simulink model "ModID_b2_R2018A"  (R2018b)
settings: Solver=VariableStepAuto  StartTime=0.0  StopTime=10.0  RelTol=1e-3
undefined symbols (not defined in the file or in its folder): par
settings Model: Creator=janneke  LastModifiedBy=janneke

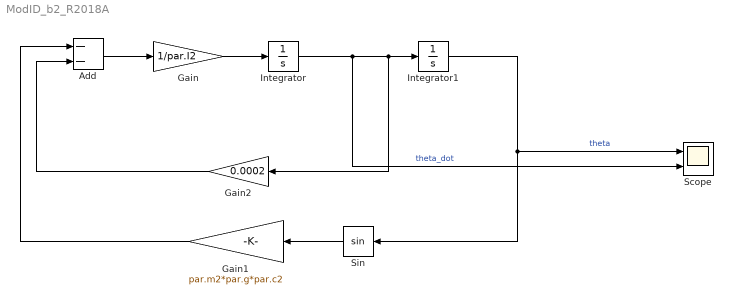
== system ModID_b2_R2018A ==
  Add : Sum  Inputs=--
  Gain : Gain  Gain=1/par.I2
  Gain1 : Gain  Gain=par.m2*par.g*par.c2
  Gain2 : Gain  Gain=0.0002
  Integrator : Integrator
  Integrator1 : Integrator  InitialCondition=-pi/2
  Scope : Scope  NumInputPorts=2
  Sin : Trigonometry
  wires:
  Integrator/1 -> Scope/2, Gain2/1, Integrator1/1  "theta_dot"
  Integrator1/1 -> Sin/1, Scope/1  "theta"
  Gain/1 -> Integrator/1
  Add/1 -> Gain/1
  Sin/1 -> Gain1/1
  Gain1/1 -> Add/1
  Gain2/1 -> Add/2
